simulink model "ROPOD_4Wheel_Tdistkinb_cntr_Code_GEN"  (R2017b)
settings: Solver=VariableStepAuto  StartTime=0.0  StopTime=10.0  RelTol=1e-3
values from neighbouring files (symbols this model uses):
  FFtheta_intia = 0    [init_model.m]
  FFxy_mass = 0*80    (= 0)    [init_model.m]
  I_fhz_dtheta_cntr = 0.3    [init_model.m]
  I_fhz_dvarphi_cntr = 0    [init_model.m]
  I_fhz_dxdy_cntr = 0.25    [init_model.m]
  K_gain_dtheta_cntr = 100    [init_model.m]
  K_gain_dvarphi_cntr = 0.03    [init_model.m]
  K_gain_dxdy_cntr = 150    [init_model.m]
  LL_wp_fhz_dtheta_cntr = 20    [init_model.m]
  LL_wp_fhz_dvarphi_cntr = 10    [init_model.m]
  LL_wp_fhz_dxdy_cntr = 20    [init_model.m]
  LL_wz_fhz_dtheta_cntr = 20    [init_model.m]
  LL_wz_fhz_dvarphi_cntr = 5    [init_model.m]
  LL_wz_fhz_dxdy_cntr = 20    [init_model.m]
  LPF_fhz_ddelta_meas = 50    [init_model.m]
  LPF_fhz_dtheta_cntr = 100    [init_model.m]
  LPF_fhz_dvarphi_cntr = 40    [init_model.m]
  LPF_fhz_dvarphi_meas = 50    [init_model.m]
  LPF_fhz_dxdy_cntr = 100    [init_model.m]
  max_hw_tau = 7.0    (= 7)    [init_model.m]
  max_ropod_acc_theta = 2.0    (= 2)    [init_model.m]
  max_ropod_acc_xy = 10.5    [init_model.m]
  max_ropod_vel_theta = 1.6    [init_model.m]
  max_ropod_vel_xy = 5.0    (= 5)    [init_model.m]
  max_sw_current = 15    [init_model.m]
  Nwheels = 4    [Jqwl_numeric_function.m]    (also in S_matrix.m; extract_kinmodel_parameters.m; init_model.m; tau_optimal_dist_vec_fun.m)
  pivot_offs_sws = 0*[3.835 3.465 2.059 0.357]    [init_model.m]
  ropod_kinmodel_pv = struct2array(ropod_kinmodel_param)    [set_ropod_KinModparams.m]
  SW_COM1_ENABLE1 = hex2dec('0001')    [init_model.m]
  SW_COM1_ENABLE2 = hex2dec('0002')    [init_model.m]
  SW_COM1_MODE_TORQUE = bitshift(hex2dec('0000'),2)    [init_model.m]
  SW_COM1_MODE_VELOCITY = bitshift(hex2dec('0002'),2)    [init_model.m]
  SW_COM1_USE_TS = hex2dec('8000')    [init_model.m]
  sw_tau_2_curr = 1/motor_physical_parameters.torqueconstant.value    [init_model.m]
  Tinit = 1*Tslot    [init_model.m]
  Ts = 0.001    [init_model.m]
undefined symbols (not defined in the file or in its folder): DiscIntNeverNeededParam
libraries: simulink x50, cstblocks x23, dspsigops x12, SOEM_EtherCAT_Lib x5
(part 1 of 4)
settings Model: Creator=cesar  LastModifiedBy=cesar
settings OptimizationCC: DefaultParameterBehavior=Inlined  UseFloatMulNetSlope=on  InlineInvariantSignals=on  EfficientFloat2IntCast=on
settings DebuggingCC: UnderSpecifiedDataTypeMsg=warning
settings HardwareCC: ProdBitPerLong=64  ProdHWDeviceType=Intel->x86-64 (Linux 64)
settings RTWCC: GenCodeOnly=on  BuildConfiguration=Faster Runs
settings GRTTargetCC: MatFileLogging=off  SupportNonFinite=off

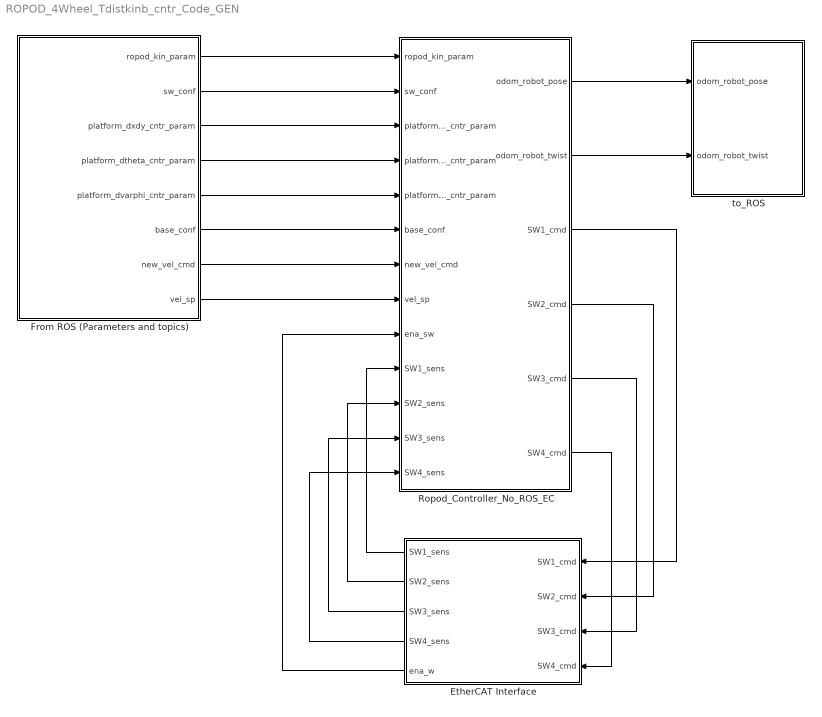
== system ROPOD_4Wheel_Tdistkinb_cntr_Code_GEN ==
  EtherCAT Interface : Subsystem
  From ROS (Parameters and topics) : Subsystem
  Ropod_Controller_No_ROS_EC : Subsystem
  to_ROS : Subsystem
  wires:
  From ROS (Parameters and topics)/1(ropod_kin_param) -> Ropod_Controller_No_ROS_EC/1(ropod_kin_param)
  Ropod_Controller_No_ROS_EC/6(SW4_cmd) -> EtherCAT Interface/4(SW4_cmd)
  From ROS (Parameters and topics)/4(platform_dtheta_cntr_param) -> Ropod_Controller_No_ROS_EC/4(platform_dtheta_cntr_param)
  Ropod_Controller_No_ROS_EC/3(SW1_cmd) -> EtherCAT Interface/1(SW1_cmd)
  From ROS (Parameters and topics)/3(platform_dxdy_cntr_param) -> Ropod_Controller_No_ROS_EC/3(platform_dxdy_cntr_param)
  Ropod_Controller_No_ROS_EC/4(SW2_cmd) -> EtherCAT Interface/2(SW2_cmd)
  EtherCAT Interface/4(SW4_sens) -> Ropod_Controller_No_ROS_EC/13(SW4_sens)
  Ropod_Controller_No_ROS_EC/2(odom_robot_twist) -> to_ROS/2(odom_robot_twist)
  Ropod_Controller_No_ROS_EC/5(SW3_cmd) -> EtherCAT Interface/3(SW3_cmd)
  From ROS (Parameters and topics)/8(vel_sp) -> Ropod_Controller_No_ROS_EC/8(vel_sp)
  From ROS (Parameters and topics)/6(base_conf) -> Ropod_Controller_No_ROS_EC/6(base_conf)
  EtherCAT Interface/1(SW1_sens) -> Ropod_Controller_No_ROS_EC/10(SW1_sens)
  From ROS (Parameters and topics)/2(sw_conf) -> Ropod_Controller_No_ROS_EC/2(sw_conf)
  From ROS (Parameters and topics)/5(platform_dvarphi_cntr_param) -> Ropod_Controller_No_ROS_EC/5(platform_dvarphi_cntr_param)
  EtherCAT Interface/2(SW2_sens) -> Ropod_Controller_No_ROS_EC/11(SW2_sens)
  EtherCAT Interface/5(ena_w) -> Ropod_Controller_No_ROS_EC/9(ena_sw)
  EtherCAT Interface/3(SW3_sens) -> Ropod_Controller_No_ROS_EC/12(SW3_sens)
  Ropod_Controller_No_ROS_EC/1(odom_robot_pose) -> to_ROS/1(odom_robot_pose)
  From ROS (Parameters and topics)/7(new_vel_cmd) -> Ropod_Controller_No_ROS_EC/7(new_vel_cmd)

== system ROPOD_4Wheel_Tdistkinb_cntr_Code_GEN/EtherCAT Interface ==
  SW1_cmd : Inport
  SW2_cmd : Inport  Port=2
  SW3_cmd : Inport  Port=3
  SW4_cmd : Inport  Port=4
  Constant : Constant  Value=[1 1 1 1]
  Display1 : Display  Commented=on
  ECAT_Interface : SOEM_EtherCAT_Lib/ECAT_Interface  Priority=0  Commented=on  IFINTERFACE=eth0  TS=Ts
      settings: SourceProductName=SOEM_EtherCAT_Lib
  Gain1 : Gain  Commented=on  OutDataTypeStr=double
  Smart_Wheel_1 : Subsystem
  Smart_Wheel_2 : Subsystem
  Smart_Wheel_3 : Subsystem
  Smart_Wheel_4 : Subsystem
  SW1_sens : Outport
  SW2_sens : Outport  Port=2
  SW3_sens : Outport  Port=3
  SW4_sens : Outport  Port=4
  ena_w : Outport  Port=5
  wires:
  Smart_Wheel_2/1(SW2_sens) -> SW2_sens/1  "SW2_sens"
  Smart_Wheel_3/1(SW3_sens) -> SW3_sens/1  "SW3_sens"
  SW4_cmd/1 -> Smart_Wheel_4/1(SW4_cmd)
  SW2_cmd/1 -> Smart_Wheel_2/1(SW2_cmd)
  SW3_cmd/1 -> Smart_Wheel_3/1(SW3_cmd)
  SW1_cmd/1 -> Smart_Wheel_1/1(SW1_cmd)
  Smart_Wheel_1/1(SW1_sens) -> SW1_sens/1  "SW1_sens"
  Smart_Wheel_4/1(SW4_sens) -> SW4_sens/1  "SW4_sens"
  ECAT_Interface/1 -> Gain1/1
  Gain1/1 -> Display1/1
  Constant/1 -> ena_w/1

== system ROPOD_4Wheel_Tdistkinb_cntr_Code_GEN/From ROS (Parameters and topics) ==
  note: doing the transformation with the angle from odometry data helps
      | to keep the robot better align during the Identification, especially because
      | we do not have any absolute reference
  Constant1 : Constant
  Controllers conf : Subsystem
  From Workspace1 : FromWorkspace  VariableName=qrefdot  SampleTime=0
  Gain1 : Gain
  ROS base conf : Subsystem
  Ropod kinematic parameters : Subsystem
  Selector1 : Selector  InputPortWidth=3  IndexOptions=Index vector (dialog)  Indices=3  OutputSizes=1
  Smart wheels conf1 : Subsystem
  rot_matrix2 : MATLAB Function  TreatAsAtomicUnit=on
  ropod_kin_param : Outport
  sw_conf : Outport  Port=2
  platform_dxdy_cntr_param : Outport  Port=3
  platform_dtheta_cntr_param : Outport  Port=4
  platform_dvarphi_cntr_param : Outport  Port=5
  base_conf : Outport  Port=6
  new_vel_cmd : Outport  Port=7
  vel_sp : Outport  Port=8
  wires:
  Controllers conf/1(platform_dxdy_cntr_param) -> platform_dxdy_cntr_param/1
  Constant1/1 -> new_vel_cmd/1
  Ropod kinematic parameters/1(ropod_kin_param) -> ropod_kin_param/1
  Gain1/1 -> vel_sp/1
  ROS base conf/1(base_conf) -> base_conf/1
  From Workspace1/1 -> Selector1/1, rot_matrix2/1(dqr_glb)
  Controllers conf/3(platform_dvarphi_cntr_param) -> platform_dvarphi_cntr_param/1
  Smart wheels conf1/1(sw_conf) -> sw_conf/1
  Controllers conf/2(platform_dtheta_cntr_param) -> platform_dtheta_cntr_param/1
  Selector1/1 -> rot_matrix2/2(theta)
  rot_matrix2/1(dqr_loc) -> Gain1/1

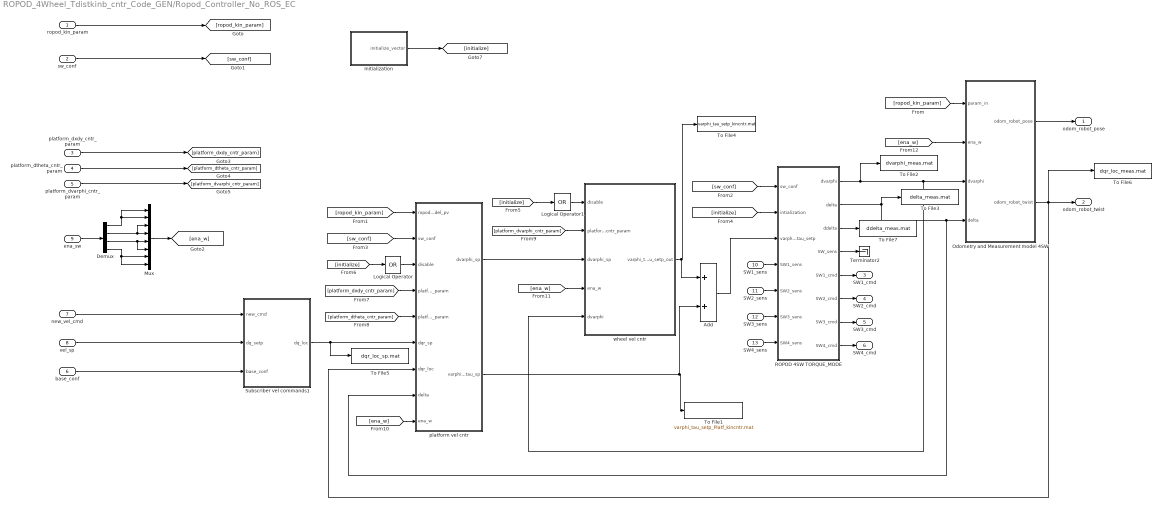
== system ROPOD_4Wheel_Tdistkinb_cntr_Code_GEN/Ropod_Controller_No_ROS_EC ==
  ropod_kin_param : Inport
  sw_conf : Inport  Port=2
  platform_dxdy_cntr_param : Inport  Port=3
  platform_dtheta_cntr_param : Inport  Port=4
  platform_dvarphi_cntr_param : Inport  Port=5
  base_conf : Inport  Port=6
  new_vel_cmd : Inport  Port=7
  vel_sp : Inport  Port=8
  ena_sw : Inport  Port=9
  SW1_sens : Inport  Port=10
  SW2_sens : Inport  Port=11
  SW3_sens : Inport  Port=12
  SW4_sens : Inport  Port=13
  Add : Sum
  Demux : Demux
  Initialization : Subsystem
  Logical Operator : Logic  Operator=OR  Inputs=1  AllPortsSameDT=off  OutDataTypeStr=boolean
  Logical Operator1 : Logic  Operator=OR  Inputs=1  AllPortsSameDT=off  OutDataTypeStr=boolean
  Mux : Mux  Inputs=8
  Odometry and Measurement model 4SW : Subsystem
  ROPOD 4SW TORQUE_MODE : Subsystem
  Subscriber vel commands1 : Subsystem
  Terminator2 : Terminator
  To File1 : ToFile  Filename=varphi_tau_setp_Platf_kincntr.mat  MatrixName=varphi_tau_setp_Platf_kincntr
  To File2 : ToFile  Filename=dvarphi_meas.mat  MatrixName=dvarphi_meas
  To File3 : ToFile  Filename=delta_meas.mat  MatrixName=delta_meas
  To File4 : ToFile  Filename=varphi_tau_setp_kincntr.mat  MatrixName=varphi_tau_setp_kincntr
  To File5 : ToFile  Filename=dqr_loc_sp.mat  MatrixName=dqr_loc_sp
  To File6 : ToFile  Filename=dqr_loc_meas.mat  MatrixName=dqr_loc_meas
  To File7 : ToFile  Filename=ddelta_meas.mat  MatrixName=ddelta_meas
  platform vel cntr : Subsystem
  wheel vel cntr : Subsystem
  odom_robot_pose : Outport
  odom_robot_twist : Outport  Port=2
  SW1_cmd : Outport  Port=3
  SW2_cmd : Outport  Port=4
  SW3_cmd : Outport  Port=5
  SW4_cmd : Outport  Port=6
  wires:
  sw_conf/1 -> [sw_conf]
  platform_dvarphi_cntr_param/1 -> [platform_dvarphi_cntr_param]
  platform_dxdy_cntr_param/1 -> [platform_dxdy_cntr_param]
  ropod_kin_param/1 -> [ropod_kin_param]
  platform_dtheta_cntr_param/1 -> [platform_dtheta_cntr_param]
  [ropod_kin_param] -> platform vel cntr/1(ropod_kinmodel_pv)
  ROPOD 4SW TORQUE_MODE/2(delta) -> To File3/1, platform vel cntr/8(delta), Odometry and Measurement model 4SW/4(delta)
  vel_sp/1 -> Subscriber vel commands1/2(dq_setp)
  ROPOD 4SW TORQUE_MODE/3(ddelta) -> To File7/1
  [initialize] -> Logical Operator/1
  wheel vel cntr/1(varphi_tau_setp_out) -> Add/1, To File4/1
  Odometry and Measurement model 4SW/2(odom_robot_twist) -> To File6/1, platform vel cntr/7(dqr_loc), odom_robot_twist/1
  [sw_conf] -> ROPOD 4SW TORQUE_MODE/1(sw_conf)
  platform vel cntr/1(dvarphi_sp) -> wheel vel cntr/3(dvarphi_sp)
  Subscriber vel commands1/1(dq_loc) -> To File5/1, platform vel cntr/6(dqr_sp)
  [platform_dvarphi_cntr_param] -> wheel vel cntr/2(platform_dxdy_cntr_param)
  base_conf/1 -> Subscriber vel commands1/3(base_conf)
  ROPOD 4SW TORQUE_MODE/1(dvarphi) -> To File2/1, wheel vel cntr/5(dvarphi), Odometry and Measurement model 4SW/3(dvarphi)
  [ropod_kin_param] -> Odometry and Measurement model 4SW/1(param_in)
  [ena_w] -> platform vel cntr/9(ena_w)
  Odometry and Measurement model 4SW/1(odom_robot_pose) -> odom_robot_pose/1
  new_vel_cmd/1 -> Subscriber vel commands1/1(new_cmd)
  [platform_dtheta_cntr_param] -> platform vel cntr/5(platform_dtheta_cntr_param)
  [initialize] -> Logical Operator1/1
  [platform_dxdy_cntr_param] -> platform vel cntr/4(platform_dxdy_cntr_param)
  [sw_conf] -> platform vel cntr/2(sw_conf)
  [initialize] -> ROPOD 4SW TORQUE_MODE/2(intialization)
  platform vel cntr/2(varphi_tau_sp) -> Add/2, To File1/1
  Initialization/1(initialize_vector) -> [initialize]
  Logical Operator/1 -> platform vel cntr/3(disable)
  Logical Operator1/1 -> wheel vel cntr/1(disable)
  [ena_w] -> wheel vel cntr/4(ena_w)
  [ena_w] -> Odometry and Measurement model 4SW/2(ena_w)
  ROPOD 4SW TORQUE_MODE/4(SW_sens) -> Terminator2/1
  ROPOD 4SW TORQUE_MODE/5(SW1_cmd) -> SW1_cmd/1
  ROPOD 4SW TORQUE_MODE/6(SW2_cmd) -> SW2_cmd/1
  ROPOD 4SW TORQUE_MODE/7(SW3_cmd) -> SW3_cmd/1
  ROPOD 4SW TORQUE_MODE/8(SW4_cmd) -> SW4_cmd/1
  SW1_sens/1 -> ROPOD 4SW TORQUE_MODE/4(SW1_sens)
  SW2_sens/1 -> ROPOD 4SW TORQUE_MODE/5(SW2_sens)
  SW3_sens/1 -> ROPOD 4SW TORQUE_MODE/6(SW3_sens)
  SW4_sens/1 -> ROPOD 4SW TORQUE_MODE/7(SW4_sens)
  ena_sw/1 -> Demux/1
  Demux/1 -> Mux/2, Mux/1
  Demux/2 -> Mux/3, Mux/4
  Demux/3 -> Mux/6, Mux/5
  Demux/4 -> Mux/7, Mux/8
  Mux/1 -> [ena_w]
  Add/1 -> ROPOD 4SW TORQUE_MODE/3(varphi_tau_setp)

== system ROPOD_4Wheel_Tdistkinb_cntr_Code_GEN/to_ROS ==
  odom_robot_pose : Inport
  odom_robot_twist : Inport  Port=2
  Terminator1 : Terminator
  Terminator2 : Terminator
  wires:
  odom_robot_pose/1 -> Terminator2/1
  odom_robot_twist/1 -> Terminator1/1

== system ROPOD_4Wheel_Tdistkinb_cntr_Code_GEN/EtherCAT Interface/Smart_Wheel_1 ==
  SW1_cmd : Inport
  Bus Creator1 : BusCreator  Inputs=40
  Bus Selector : BusSelector  OutputSignals=command1,command2,setpoint1,setpoint2,limit1_p,limit1_n,limit2_p,limit2_n,timestamp
  ec_ROPOD_SmartWheel : SOEM_EtherCAT_Lib/ec_ROPOD_SmartWheel  link_id=1
      settings: SourceProductName=SOEM_EtherCAT_Lib
  SW1_sens : Outport
  wires:
  Bus Creator1/1 -> SW1_sens/1
  ec_ROPOD_SmartWheel/21 -> Bus Creator1/21  "current_2_u"
  ec_ROPOD_SmartWheel/3 -> Bus Creator1/3  "sensor_ts"
  ec_ROPOD_SmartWheel/34 -> Bus Creator1/34  "accel_y"
  ec_ROPOD_SmartWheel/29 -> Bus Creator1/29  "encoder_pivot"
  ec_ROPOD_SmartWheel/18 -> Bus Creator1/18  "velocity_2"
  ec_ROPOD_SmartWheel/19 -> Bus Creator1/19  "current_2_d"
  ec_ROPOD_SmartWheel/14 -> Bus Creator1/14  "voltage_1_v"
  ec_ROPOD_SmartWheel/6 -> Bus Creator1/6  "velocity_1"
  ec_ROPOD_SmartWheel/12 -> Bus Creator1/12  "voltage_1"
  ec_ROPOD_SmartWheel/35 -> Bus Creator1/35  "accel_z"
  ec_ROPOD_SmartWheel/2 -> Bus Creator1/2  "status2"
  ec_ROPOD_SmartWheel/1 -> Bus Creator1/1  "status1"
  ec_ROPOD_SmartWheel/22 -> Bus Creator1/22  "current_2_v"
  ec_ROPOD_SmartWheel/25 -> Bus Creator1/25  "voltage_2_u"
  ec_ROPOD_SmartWheel/24 -> Bus Creator1/24  "voltage_2"
  ec_ROPOD_SmartWheel/15 -> Bus Creator1/15  "voltage_1_w"
  ec_ROPOD_SmartWheel/9 -> Bus Creator1/9  "current_1_u"
  ec_ROPOD_SmartWheel/28 -> Bus Creator1/28  "temperature_2"
  ec_ROPOD_SmartWheel/37 -> Bus Creator1/37  "gyro_y"
  ec_ROPOD_SmartWheel/20 -> Bus Creator1/20  "current_2_q"
  ec_ROPOD_SmartWheel/38 -> Bus Creator1/38  "gyro_z"
  ec_ROPOD_SmartWheel/13 -> Bus Creator1/13  "voltage_1_u"
  ec_ROPOD_SmartWheel/27 -> Bus Creator1/27  "voltage_2_w"
  ec_ROPOD_SmartWheel/7 -> Bus Creator1/7  "current_1_d"
  ec_ROPOD_SmartWheel/5 -> Bus Creator1/5  "encoder_1"
  ec_ROPOD_SmartWheel/36 -> Bus Creator1/36  "gyro_x"
  ec_ROPOD_SmartWheel/23 -> Bus Creator1/23  "current_2_w"
  ec_ROPOD_SmartWheel/4 -> Bus Creator1/4  "setpoint_ts"
  ec_ROPOD_SmartWheel/17 -> Bus Creator1/17  "encoder_2"
  ec_ROPOD_SmartWheel/11 -> Bus Creator1/11  "current_1_w"
  ec_ROPOD_SmartWheel/40 -> Bus Creator1/40  "pressure"
  ec_ROPOD_SmartWheel/30 -> Bus Creator1/30  "velocity_pivot"
  ec_ROPOD_SmartWheel/10 -> Bus Creator1/10  "current_1_v"
  ec_ROPOD_SmartWheel/39 -> Bus Creator1/39  "temperature_imu"
  ec_ROPOD_SmartWheel/16 -> Bus Creator1/16  "temperature_1"
  ec_ROPOD_SmartWheel/33 -> Bus Creator1/33  "accel_x"
  ec_ROPOD_SmartWheel/26 -> Bus Creator1/26  "voltage_2_v"
  ec_ROPOD_SmartWheel/8 -> Bus Creator1/8  "current_1_q"
  ec_ROPOD_SmartWheel/31 -> Bus Creator1/31  "voltage_bus"
  ec_ROPOD_SmartWheel/32 -> Bus Creator1/32  "imu_ts"
  SW1_cmd/1 -> Bus Selector/1
  Bus Selector/1 -> ec_ROPOD_SmartWheel/1  "<command1>"
  Bus Selector/2 -> ec_ROPOD_SmartWheel/2  "<command2>"
  Bus Selector/3 -> ec_ROPOD_SmartWheel/3  "<setpoint1>"
  Bus Selector/4 -> ec_ROPOD_SmartWheel/4  "<setpoint2>"
  Bus Selector/5 -> ec_ROPOD_SmartWheel/5  "<limit1_p>"
  Bus Selector/6 -> ec_ROPOD_SmartWheel/6  "<limit1_n>"
  Bus Selector/7 -> ec_ROPOD_SmartWheel/7  "<limit2_p>"
  Bus Selector/8 -> ec_ROPOD_SmartWheel/8  "<limit2_n>"
  Bus Selector/9 -> ec_ROPOD_SmartWheel/9  "<timestamp>"

== system ROPOD_4Wheel_Tdistkinb_cntr_Code_GEN/EtherCAT Interface/Smart_Wheel_2 ==
  SW2_cmd : Inport
  Bus Creator1 : BusCreator  Inputs=40
  Bus Selector : BusSelector  OutputSignals=command1,command2,setpoint1,setpoint2,limit1_p,limit1_n,limit2_p,limit2_n,timestamp
  ec_ROPOD_SmartWheel : SOEM_EtherCAT_Lib/ec_ROPOD_SmartWheel  link_id=2
      settings: SourceProductName=SOEM_EtherCAT_Lib
  SW2_sens : Outport
  wires:
  Bus Selector/9 -> ec_ROPOD_SmartWheel/9  "<timestamp>"
  Bus Selector/8 -> ec_ROPOD_SmartWheel/8  "<limit2_n>"
  Bus Selector/7 -> ec_ROPOD_SmartWheel/7  "<limit2_p>"
  Bus Selector/6 -> ec_ROPOD_SmartWheel/6  "<limit1_n>"
  Bus Selector/5 -> ec_ROPOD_SmartWheel/5  "<limit1_p>"
  Bus Selector/4 -> ec_ROPOD_SmartWheel/4  "<setpoint2>"
  Bus Selector/3 -> ec_ROPOD_SmartWheel/3  "<setpoint1>"
  Bus Selector/2 -> ec_ROPOD_SmartWheel/2  "<command2>"
  Bus Selector/1 -> ec_ROPOD_SmartWheel/1  "<command1>"
  SW2_cmd/1 -> Bus Selector/1
  ec_ROPOD_SmartWheel/32 -> Bus Creator1/32  "imu_ts"
  ec_ROPOD_SmartWheel/31 -> Bus Creator1/31  "voltage_bus"
  ec_ROPOD_SmartWheel/8 -> Bus Creator1/8  "current_1_q"
  ec_ROPOD_SmartWheel/26 -> Bus Creator1/26  "voltage_2_v"
  ec_ROPOD_SmartWheel/33 -> Bus Creator1/33  "accel_x"
  ec_ROPOD_SmartWheel/16 -> Bus Creator1/16  "temperature_1"
  ec_ROPOD_SmartWheel/39 -> Bus Creator1/39  "temperature_imu"
  ec_ROPOD_SmartWheel/10 -> Bus Creator1/10  "current_1_v"
  ec_ROPOD_SmartWheel/30 -> Bus Creator1/30  "velocity_pivot"
  ec_ROPOD_SmartWheel/40 -> Bus Creator1/40  "pressure"
  ec_ROPOD_SmartWheel/11 -> Bus Creator1/11  "current_1_w"
  ec_ROPOD_SmartWheel/17 -> Bus Creator1/17  "encoder_2"
  ec_ROPOD_SmartWheel/4 -> Bus Creator1/4  "setpoint_ts"
  ec_ROPOD_SmartWheel/23 -> Bus Creator1/23  "current_2_w"
  ec_ROPOD_SmartWheel/36 -> Bus Creator1/36  "gyro_x"
  ec_ROPOD_SmartWheel/5 -> Bus Creator1/5  "encoder_1"
  ec_ROPOD_SmartWheel/7 -> Bus Creator1/7  "current_1_d"
  ec_ROPOD_SmartWheel/27 -> Bus Creator1/27  "voltage_2_w"
  ec_ROPOD_SmartWheel/13 -> Bus Creator1/13  "voltage_1_u"
  ec_ROPOD_SmartWheel/38 -> Bus Creator1/38  "gyro_z"
  ec_ROPOD_SmartWheel/20 -> Bus Creator1/20  "current_2_q"
  ec_ROPOD_SmartWheel/37 -> Bus Creator1/37  "gyro_y"
  ec_ROPOD_SmartWheel/28 -> Bus Creator1/28  "temperature_2"
  ec_ROPOD_SmartWheel/9 -> Bus Creator1/9  "current_1_u"
  ec_ROPOD_SmartWheel/15 -> Bus Creator1/15  "voltage_1_w"
  ec_ROPOD_SmartWheel/24 -> Bus Creator1/24  "voltage_2"
  ec_ROPOD_SmartWheel/25 -> Bus Creator1/25  "voltage_2_u"
  ec_ROPOD_SmartWheel/22 -> Bus Creator1/22  "current_2_v"
  ec_ROPOD_SmartWheel/1 -> Bus Creator1/1  "status1"
  ec_ROPOD_SmartWheel/2 -> Bus Creator1/2  "status2"
  ec_ROPOD_SmartWheel/35 -> Bus Creator1/35  "accel_z"
  ec_ROPOD_SmartWheel/12 -> Bus Creator1/12  "voltage_1"
  ec_ROPOD_SmartWheel/6 -> Bus Creator1/6  "velocity_1"
  ec_ROPOD_SmartWheel/14 -> Bus Creator1/14  "voltage_1_v"
  ec_ROPOD_SmartWheel/19 -> Bus Creator1/19  "current_2_d"
  ec_ROPOD_SmartWheel/18 -> Bus Creator1/18  "velocity_2"
  ec_ROPOD_SmartWheel/29 -> Bus Creator1/29  "encoder_pivot"
  ec_ROPOD_SmartWheel/34 -> Bus Creator1/34  "accel_y"
  ec_ROPOD_SmartWheel/3 -> Bus Creator1/3  "sensor_ts"
  ec_ROPOD_SmartWheel/21 -> Bus Creator1/21  "current_2_u"
  Bus Creator1/1 -> SW2_sens/1

== system ROPOD_4Wheel_Tdistkinb_cntr_Code_GEN/EtherCAT Interface/Smart_Wheel_3 ==
  SW3_cmd : Inport
  Bus Creator1 : BusCreator  Inputs=40
  Bus Selector : BusSelector  OutputSignals=command1,command2,setpoint1,setpoint2,limit1_p,limit1_n,limit2_p,limit2_n,timestamp
  ec_ROPOD_SmartWheel : SOEM_EtherCAT_Lib/ec_ROPOD_SmartWheel  link_id=3
      settings: SourceProductName=SOEM_EtherCAT_Lib
  SW3_sens : Outport
  wires:
  Bus Creator1/1 -> SW3_sens/1
  ec_ROPOD_SmartWheel/21 -> Bus Creator1/21  "current_2_u"
  ec_ROPOD_SmartWheel/3 -> Bus Creator1/3  "sensor_ts"
  ec_ROPOD_SmartWheel/34 -> Bus Creator1/34  "accel_y"
  ec_ROPOD_SmartWheel/29 -> Bus Creator1/29  "encoder_pivot"
  ec_ROPOD_SmartWheel/18 -> Bus Creator1/18  "velocity_2"
  ec_ROPOD_SmartWheel/19 -> Bus Creator1/19  "current_2_d"
  ec_ROPOD_SmartWheel/14 -> Bus Creator1/14  "voltage_1_v"
  ec_ROPOD_SmartWheel/6 -> Bus Creator1/6  "velocity_1"
  ec_ROPOD_SmartWheel/12 -> Bus Creator1/12  "voltage_1"
  ec_ROPOD_SmartWheel/35 -> Bus Creator1/35  "accel_z"
  ec_ROPOD_SmartWheel/2 -> Bus Creator1/2  "status2"
  ec_ROPOD_SmartWheel/1 -> Bus Creator1/1  "status1"
  ec_ROPOD_SmartWheel/22 -> Bus Creator1/22  "current_2_v"
  ec_ROPOD_SmartWheel/25 -> Bus Creator1/25  "voltage_2_u"
  ec_ROPOD_SmartWheel/24 -> Bus Creator1/24  "voltage_2"
  ec_ROPOD_SmartWheel/15 -> Bus Creator1/15  "voltage_1_w"
  ec_ROPOD_SmartWheel/9 -> Bus Creator1/9  "current_1_u"
  ec_ROPOD_SmartWheel/28 -> Bus Creator1/28  "temperature_2"
  ec_ROPOD_SmartWheel/37 -> Bus Creator1/37  "gyro_y"
  ec_ROPOD_SmartWheel/20 -> Bus Creator1/20  "current_2_q"
  ec_ROPOD_SmartWheel/38 -> Bus Creator1/38  "gyro_z"
  ec_ROPOD_SmartWheel/13 -> Bus Creator1/13  "voltage_1_u"
  ec_ROPOD_SmartWheel/27 -> Bus Creator1/27  "voltage_2_w"
  ec_ROPOD_SmartWheel/7 -> Bus Creator1/7  "current_1_d"
  ec_ROPOD_SmartWheel/5 -> Bus Creator1/5  "encoder_1"
  ec_ROPOD_SmartWheel/36 -> Bus Creator1/36  "gyro_x"
  ec_ROPOD_SmartWheel/23 -> Bus Creator1/23  "current_2_w"
  ec_ROPOD_SmartWheel/4 -> Bus Creator1/4  "setpoint_ts"
  ec_ROPOD_SmartWheel/17 -> Bus Creator1/17  "encoder_2"
  ec_ROPOD_SmartWheel/11 -> Bus Creator1/11  "current_1_w"
  ec_ROPOD_SmartWheel/40 -> Bus Creator1/40  "pressure"
  ec_ROPOD_SmartWheel/30 -> Bus Creator1/30  "velocity_pivot"
  ec_ROPOD_SmartWheel/10 -> Bus Creator1/10  "current_1_v"
  ec_ROPOD_SmartWheel/39 -> Bus Creator1/39  "temperature_imu"
  ec_ROPOD_SmartWheel/16 -> Bus Creator1/16  "temperature_1"
  ec_ROPOD_SmartWheel/33 -> Bus Creator1/33  "accel_x"
  ec_ROPOD_SmartWheel/26 -> Bus Creator1/26  "voltage_2_v"
  ec_ROPOD_SmartWheel/8 -> Bus Creator1/8  "current_1_q"
  ec_ROPOD_SmartWheel/31 -> Bus Creator1/31  "voltage_bus"
  ec_ROPOD_SmartWheel/32 -> Bus Creator1/32  "imu_ts"
  SW3_cmd/1 -> Bus Selector/1
  Bus Selector/1 -> ec_ROPOD_SmartWheel/1  "<command1>"
  Bus Selector/2 -> ec_ROPOD_SmartWheel/2  "<command2>"
  Bus Selector/3 -> ec_ROPOD_SmartWheel/3  "<setpoint1>"
  Bus Selector/4 -> ec_ROPOD_SmartWheel/4  "<setpoint2>"
  Bus Selector/5 -> ec_ROPOD_SmartWheel/5  "<limit1_p>"
  Bus Selector/6 -> ec_ROPOD_SmartWheel/6  "<limit1_n>"
  Bus Selector/7 -> ec_ROPOD_SmartWheel/7  "<limit2_p>"
  Bus Selector/8 -> ec_ROPOD_SmartWheel/8  "<limit2_n>"
  Bus Selector/9 -> ec_ROPOD_SmartWheel/9  "<timestamp>"

== system ROPOD_4Wheel_Tdistkinb_cntr_Code_GEN/EtherCAT Interface/Smart_Wheel_4 ==
  SW4_cmd : Inport
  Bus Creator1 : BusCreator  Inputs=40
  Bus Selector : BusSelector  OutputSignals=command1,command2,setpoint1,setpoint2,limit1_p,limit1_n,limit2_p,limit2_n,timestamp
  ec_ROPOD_SmartWheel : SOEM_EtherCAT_Lib/ec_ROPOD_SmartWheel  link_id=4
      settings: SourceProductName=SOEM_EtherCAT_Lib
  SW4_sens : Outport
  wires:
  Bus Selector/9 -> ec_ROPOD_SmartWheel/9  "<timestamp>"
  Bus Selector/8 -> ec_ROPOD_SmartWheel/8  "<limit2_n>"
  Bus Selector/7 -> ec_ROPOD_SmartWheel/7  "<limit2_p>"
  Bus Selector/6 -> ec_ROPOD_SmartWheel/6  "<limit1_n>"
  Bus Selector/5 -> ec_ROPOD_SmartWheel/5  "<limit1_p>"
  Bus Selector/4 -> ec_ROPOD_SmartWheel/4  "<setpoint2>"
  Bus Selector/3 -> ec_ROPOD_SmartWheel/3  "<setpoint1>"
  Bus Selector/2 -> ec_ROPOD_SmartWheel/2  "<command2>"
  Bus Selector/1 -> ec_ROPOD_SmartWheel/1  "<command1>"
  SW4_cmd/1 -> Bus Selector/1
  ec_ROPOD_SmartWheel/32 -> Bus Creator1/32  "imu_ts"
  ec_ROPOD_SmartWheel/31 -> Bus Creator1/31  "voltage_bus"
  ec_ROPOD_SmartWheel/8 -> Bus Creator1/8  "current_1_q"
  ec_ROPOD_SmartWheel/26 -> Bus Creator1/26  "voltage_2_v"
  ec_ROPOD_SmartWheel/33 -> Bus Creator1/33  "accel_x"
  ec_ROPOD_SmartWheel/16 -> Bus Creator1/16  "temperature_1"
  ec_ROPOD_SmartWheel/39 -> Bus Creator1/39  "temperature_imu"
  ec_ROPOD_SmartWheel/10 -> Bus Creator1/10  "current_1_v"
  ec_ROPOD_SmartWheel/30 -> Bus Creator1/30  "velocity_pivot"
  ec_ROPOD_SmartWheel/40 -> Bus Creator1/40  "pressure"
  ec_ROPOD_SmartWheel/11 -> Bus Creator1/11  "current_1_w"
  ec_ROPOD_SmartWheel/17 -> Bus Creator1/17  "encoder_2"
  ec_ROPOD_SmartWheel/4 -> Bus Creator1/4  "setpoint_ts"
  ec_ROPOD_SmartWheel/23 -> Bus Creator1/23  "current_2_w"
  ec_ROPOD_SmartWheel/36 -> Bus Creator1/36  "gyro_x"
  ec_ROPOD_SmartWheel/5 -> Bus Creator1/5  "encoder_1"
  ec_ROPOD_SmartWheel/7 -> Bus Creator1/7  "current_1_d"
  ec_ROPOD_SmartWheel/27 -> Bus Creator1/27  "voltage_2_w"
  ec_ROPOD_SmartWheel/13 -> Bus Creator1/13  "voltage_1_u"
  ec_ROPOD_SmartWheel/38 -> Bus Creator1/38  "gyro_z"
  ec_ROPOD_SmartWheel/20 -> Bus Creator1/20  "current_2_q"
  ec_ROPOD_SmartWheel/37 -> Bus Creator1/37  "gyro_y"
  ec_ROPOD_SmartWheel/28 -> Bus Creator1/28  "temperature_2"
  ec_ROPOD_SmartWheel/9 -> Bus Creator1/9  "current_1_u"
  ec_ROPOD_SmartWheel/15 -> Bus Creator1/15  "voltage_1_w"
  ec_ROPOD_SmartWheel/24 -> Bus Creator1/24  "voltage_2"
  ec_ROPOD_SmartWheel/25 -> Bus Creator1/25  "voltage_2_u"
  ec_ROPOD_SmartWheel/22 -> Bus Creator1/22  "current_2_v"
  ec_ROPOD_SmartWheel/1 -> Bus Creator1/1  "status1"
  ec_ROPOD_SmartWheel/2 -> Bus Creator1/2  "status2"
  ec_ROPOD_SmartWheel/35 -> Bus Creator1/35  "accel_z"
  ec_ROPOD_SmartWheel/12 -> Bus Creator1/12  "voltage_1"
  ec_ROPOD_SmartWheel/6 -> Bus Creator1/6  "velocity_1"
  ec_ROPOD_SmartWheel/14 -> Bus Creator1/14  "voltage_1_v"
  ec_ROPOD_SmartWheel/19 -> Bus Creator1/19  "current_2_d"
  ec_ROPOD_SmartWheel/18 -> Bus Creator1/18  "velocity_2"
  ec_ROPOD_SmartWheel/29 -> Bus Creator1/29  "encoder_pivot"
  ec_ROPOD_SmartWheel/34 -> Bus Creator1/34  "accel_y"
  ec_ROPOD_SmartWheel/3 -> Bus Creator1/3  "sensor_ts"
  ec_ROPOD_SmartWheel/21 -> Bus Creator1/21  "current_2_u"
  Bus Creator1/1 -> SW4_sens/1

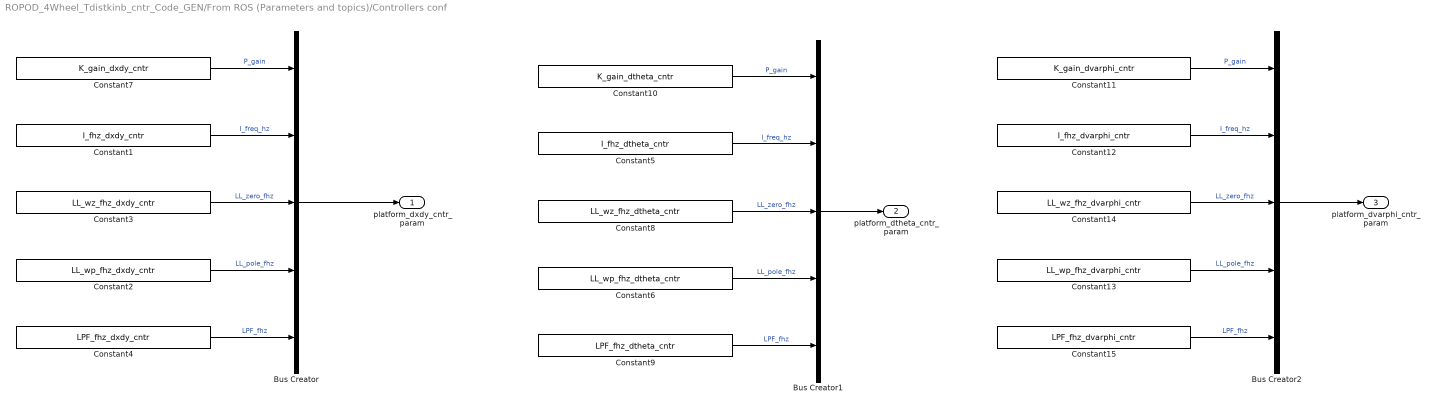
== system ROPOD_4Wheel_Tdistkinb_cntr_Code_GEN/From ROS (Parameters and topics)/Controllers conf ==
  Bus Creator : BusCreator  Inputs=5
  Bus Creator1 : BusCreator  Inputs=5
  Bus Creator2 : BusCreator  Inputs=5
  Constant1 : Constant  Value=I_fhz_dxdy_cntr
  Constant10 : Constant  Value=K_gain_dtheta_cntr
  Constant11 : Constant  Value=K_gain_dvarphi_cntr
  Constant12 : Constant  Value=I_fhz_dvarphi_cntr
  Constant13 : Constant  Value=LL_wp_fhz_dvarphi_cntr
  Constant14 : Constant  Value=LL_wz_fhz_dvarphi_cntr
  Constant15 : Constant  Value=LPF_fhz_dvarphi_cntr
  Constant2 : Constant  Value=LL_wp_fhz_dxdy_cntr
  Constant3 : Constant  Value=LL_wz_fhz_dxdy_cntr
  Constant4 : Constant  Value=LPF_fhz_dxdy_cntr
  Constant5 : Constant  Value=I_fhz_dtheta_cntr
  Constant6 : Constant  Value=LL_wp_fhz_dtheta_cntr
  Constant7 : Constant  Value=K_gain_dxdy_cntr
  Constant8 : Constant  Value=LL_wz_fhz_dtheta_cntr
  Constant9 : Constant  Value=LPF_fhz_dtheta_cntr
  platform_dxdy_cntr_param : Outport
  platform_dtheta_cntr_param : Outport  Port=2
  platform_dvarphi_cntr_param : Outport  Port=3
  wires:
  Constant2/1 -> Bus Creator/4  "LL_pole_fhz"
  Constant4/1 -> Bus Creator/5  "LPF_fhz"
  Bus Creator/1 -> platform_dxdy_cntr_param/1
  Constant1/1 -> Bus Creator/2  "I_freq_hz"
  Constant3/1 -> Bus Creator/3  "LL_zero_fhz"
  Constant7/1 -> Bus Creator/1  "P_gain"
  Bus Creator1/1 -> platform_dtheta_cntr_param/1
  Bus Creator2/1 -> platform_dvarphi_cntr_param/1
  Constant5/1 -> Bus Creator1/2  "I_freq_hz"
  Constant6/1 -> Bus Creator1/4  "LL_pole_fhz"
  Constant10/1 -> Bus Creator1/1  "P_gain"
  Constant8/1 -> Bus Creator1/3  "LL_zero_fhz"
  Constant9/1 -> Bus Creator1/5  "LPF_fhz"
  Constant15/1 -> Bus Creator2/5  "LPF_fhz"
  Constant12/1 -> Bus Creator2/2  "I_freq_hz"
  Constant14/1 -> Bus Creator2/3  "LL_zero_fhz"
  Constant11/1 -> Bus Creator2/1  "P_gain"
  Constant13/1 -> Bus Creator2/4  "LL_pole_fhz"

== system ROPOD_4Wheel_Tdistkinb_cntr_Code_GEN/From ROS (Parameters and topics)/ROS base conf ==
  Bus Creator : BusCreator  Inputs=4
  max_ropod_acc_theta : Constant  Value=max_ropod_acc_theta
  max_ropod_acc_xy : Constant  Value=max_ropod_acc_xy
  max_ropod_vel_theta : Constant  Value=max_ropod_vel_theta
  max_ropod_vel_xy : Constant  Value=max_ropod_vel_xy
  base_conf : Outport
  wires:
  max_ropod_acc_xy/1 -> Bus Creator/2  "max_acc_xy"
  max_ropod_vel_xy/1 -> Bus Creator/1  "max_vel_xy"
  Bus Creator/1 -> base_conf/1
  max_ropod_acc_theta/1 -> Bus Creator/4  "max_acc_theta"
  max_ropod_vel_theta/1 -> Bus Creator/3  "max_vel_theta"

== system ROPOD_4Wheel_Tdistkinb_cntr_Code_GEN/From ROS (Parameters and topics)/Ropod kinematic parameters ==
  ropod_kinmodel_pv : Constant  Value=ropod_kinmodel_pv
  ropod_kin_param : Outport
  wires:
  ropod_kinmodel_pv/1 -> ropod_kin_param/1

== system ROPOD_4Wheel_Tdistkinb_cntr_Code_GEN/From ROS (Parameters and topics)/Smart wheels conf1 ==
  Bus Creator : BusCreator  Inputs=8
  LPF_fhz_ddelta_meas : Constant  Value=LPF_fhz_ddelta_meas
  LPF_fhz_dvarphi_meas : Constant  Value=LPF_fhz_dvarphi_meas
  enable : Constant
  max_current : Constant  Value=max_sw_current
  pivot_offset_sw1 : Constant  Value=pivot_offs_sws(1)
  pivot_offset_sw2 : Constant  Value=pivot_offs_sws(2)
  pivot_offset_sw3 : Constant  Value=pivot_offs_sws(3)
  pivot_offset_sw4 : Constant  Value=pivot_offs_sws(4)
  sw_conf : Outport
  wires:
  enable/1 -> Bus Creator/1  "enable"
  Bus Creator/1 -> sw_conf/1
  max_current/1 -> Bus Creator/2  "max_current"
  pivot_offset_sw1/1 -> Bus Creator/3  "pivot_offs_sw1"
  pivot_offset_sw2/1 -> Bus Creator/4  "pivot_offs_sw2"
  pivot_offset_sw3/1 -> Bus Creator/5  "pivot_offs_sw3"
  pivot_offset_sw4/1 -> Bus Creator/6  "pivot_offs_sw4"
  LPF_fhz_dvarphi_meas/1 -> Bus Creator/7  "dvarphi_LPF_fhz"
  LPF_fhz_ddelta_meas/1 -> Bus Creator/8  "ddelta_LPF_fhz"

== system ROPOD_4Wheel_Tdistkinb_cntr_Code_GEN/Ropod_Controller_No_ROS_EC/Initialization ==
  note: Allow Tinit/Nwheels seconds for initialization per wheel
  Allow Tinit seconds for initialization : simulink/Logic and Bit Operations/Compare To Constant  relop=<  const=Tinit  OutDataTypeStr=boolean
  Digital Clock : DigitalClock  SampleTime=Ts
  Logical Operator : Logic  AllPortsSameDT=off  OutDataTypeStr=boolean
  Logical Operator1 : Logic  Operator=NOT  AllPortsSameDT=off  OutDataTypeStr=boolean
  Logical Operator2 : Logic  Operator=NOT  AllPortsSameDT=off  OutDataTypeStr=boolean
  Logical Operator3 : Logic  AllPortsSameDT=off  OutDataTypeStr=boolean
  Logical Operator4 : Logic  Operator=NOT  AllPortsSameDT=off  OutDataTypeStr=boolean
  Logical Operator5 : Logic  AllPortsSameDT=off  OutDataTypeStr=boolean
  Logical Operator{6..9} (4 alike) : Logic  Operator=OR  AllPortsSameDT=off  OutDataTypeStr=boolean
  Manual Switch : ManualSwitch  CurrentSetting=0
  Mux : Mux
  Mux1 : Mux
  comp : simulink/Logic and Bit Operations/Compare To Constant  relop=<  const=Tinit/Nwheels  OutDataTypeStr=boolean
  comp1 : simulink/Logic and Bit Operations/Compare To Constant  relop=<  const=2*Tinit/Nwheels  OutDataTypeStr=boolean
  comp2 : simulink/Logic and Bit Operations/Compare To Constant  relop=<  const=3*Tinit/Nwheels  OutDataTypeStr=boolean
  comp3 : simulink/Logic and Bit Operations/Compare To Constant  relop=<  const=4*Tinit/Nwheels  OutDataTypeStr=boolean
  initialize_vector : Outport
  wires:
  comp3/1 -> Logical Operator5/2
  Logical Operator2/1 -> Logical Operator3/1
  Logical Operator1/1 -> Logical Operator/1
  Logical Operator4/1 -> Logical Operator5/1
  comp/1 -> Logical Operator6/1, Mux/1, Logical Operator1/1
  comp1/1 -> Logical Operator2/1, Logical Operator/2
  comp2/1 -> Logical Operator4/1, Logical Operator3/2
  Digital Clock/1 -> Allow Tinit seconds for initialization/1, comp3/1, comp2/1, comp1/1, comp/1
  Logical Operator/1 -> Logical Operator7/1, Mux/2
  Logical Operator3/1 -> Logical Operator8/1, Mux/3
  Logical Operator5/1 -> Logical Operator9/1, Mux/4
  Logical Operator6/1 -> Mux1/1
  Logical Operator7/1 -> Mux1/2
  Logical Operator8/1 -> Mux1/3
  Logical Operator9/1 -> Mux1/4
  Allow Tinit seconds for initialization/1 -> Logical Operator6/2, Logical Operator7/2, Logical Operator8/2, Logical Operator9/2
  Manual Switch/1 -> initialize_vector/1
  Mux/1 -> Manual Switch/1
  Mux1/1 -> Manual Switch/2

== system ROPOD_4Wheel_Tdistkinb_cntr_Code_GEN/Ropod_Controller_No_ROS_EC/Odometry and Measurement model 4SW ==
  note: This output is only useful when using ros
      | This data is fed to /odom/pose
  note: This part is in global coordinates
  note: This part is in local coordinates
  param_in : Inport
  ena_w : Inport  Port=2
  dvarphi : Inport  Port=3
  delta : Inport  Port=4
  Discrete-Time Integrator : DiscreteIntegrator  InitialConditionSetting=State (most efficient)  SampleTime=Ts  ICPrevOutput=DiscIntNeverNeededParam  ICPrevScaledInput=DiscIntNeverNeededParam
  Jqwl_numeric : MATLAB Function  TreatAsAtomicUnit=on
  Selector3 : Selector  IndexMode=Zero-based  InputPortWidth=3  IndexOptions=Index vector (dialog)  Indices=2  OutputSizes=1
  Signal Specification : SignalSpecification  Dimensions=[3 1]
  pos_rot_matrix : MATLAB Function  TreatAsAtomicUnit=on
  odom_robot_pose : Outport
  odom_robot_twist : Outport  Port=2
  wires:
  Jqwl_numeric/1(v) -> Signal Specification/1
  param_in/1 -> Jqwl_numeric/1(ropod_kinmodel_param_vec)
  delta/1 -> Jqwl_numeric/2(delta)
  Signal Specification/1 -> pos_rot_matrix/1(dqr_loc), odom_robot_twist/1
  Selector3/1 -> pos_rot_matrix/2(theta_odom)
  pos_rot_matrix/1(dqr_glb) -> Discrete-Time Integrator/1
  Discrete-Time Integrator/1 -> odom_robot_pose/1, Selector3/1
  dvarphi/1 -> Jqwl_numeric/3(dvarphi)
  ena_w/1 -> Jqwl_numeric/4(ena_w)

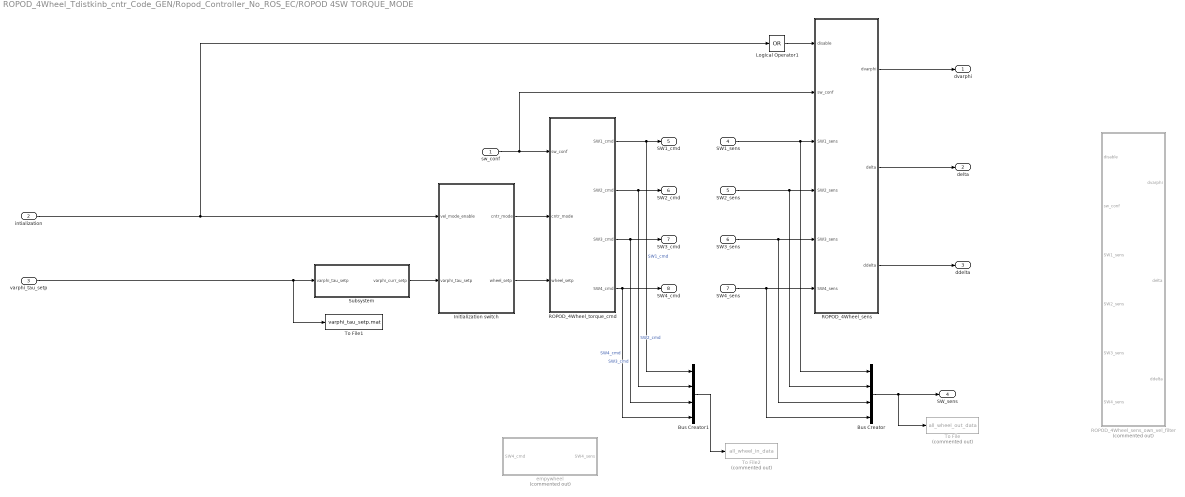
== system ROPOD_4Wheel_Tdistkinb_cntr_Code_GEN/Ropod_Controller_No_ROS_EC/ROPOD 4SW TORQUE_MODE ==
  sw_conf : Inport
  intialization : Inport  Port=2
  varphi_tau_setp : Inport  Port=3
  SW1_sens : Inport  Port=4
  SW2_sens : Inport  Port=5
  SW3_sens : Inport  Port=6
  SW4_sens : Inport  Port=7
  Bus Creator : BusCreator  Inputs=4
  Bus Creator1 : BusCreator  Inputs=4
  Initialization switch : Subsystem
  Logical Operator1 : Logic  Operator=OR  Inputs=1  AllPortsSameDT=off  OutDataTypeStr=boolean
  ROPOD_4Wheel_sens : Subsystem
  ROPOD_4Wheel_sens_own_vel_filter : Subsystem  Commented=on
  ROPOD_4Wheel_torque_cmd : Subsystem
  Subsystem : Subsystem
  To File : ToFile  Commented=on  Filename=all_wheel_out_data  MatrixName=all_wheel_out_data
  To File1 : ToFile  Filename=varphi_tau_setp.mat  MatrixName=varphi_tau_setp
  To File2 : ToFile  Commented=on  Filename=all_wheel_in_data  MatrixName=all_wheel_in_data
  empywheel : Subsystem  Commented=on
  dvarphi : Outport
  delta : Outport  Port=2
  ddelta : Outport  Port=3
  SW_sens : Outport  Port=4
  SW1_cmd : Outport  Port=5
  SW2_cmd : Outport  Port=6
  SW3_cmd : Outport  Port=7
  SW4_cmd : Outport  Port=8
  wires:
  ROPOD_4Wheel_sens/2(delta) -> delta/1
  ROPOD_4Wheel_sens/1(dvarphi) -> dvarphi/1
  ROPOD_4Wheel_sens/3(ddelta) -> ddelta/1
  ROPOD_4Wheel_torque_cmd/4(SW4_cmd) -> SW4_cmd/1, Bus Creator1/4  "SW4_cmd"
  ROPOD_4Wheel_torque_cmd/1(SW1_cmd) -> SW1_cmd/1, Bus Creator1/1  "SW1_cmd"
  ROPOD_4Wheel_torque_cmd/3(SW3_cmd) -> SW3_cmd/1, Bus Creator1/3  "SW3_cmd"
  sw_conf/1 -> ROPOD_4Wheel_sens/2(sw_conf), ROPOD_4Wheel_torque_cmd/1(sw_conf)
  ROPOD_4Wheel_torque_cmd/2(SW2_cmd) -> SW2_cmd/1, Bus Creator1/2  "SW2_cmd"
  Bus Creator/1 -> To File/1, SW_sens/1
  Initialization switch/1(cntr_mode) -> ROPOD_4Wheel_torque_cmd/2(cntr_mode)
  Initialization switch/2(wheel_setp) -> ROPOD_4Wheel_torque_cmd/3(wheel_setp)
  Subsystem/1(varphi_curr_setp) -> Initialization switch/2(varphi_tau_setp)
  varphi_tau_setp/1 -> To File1/1, Subsystem/1(varphi_tau_setp)
  intialization/1 -> Initialization switch/1(vel_mode_enable), Logical Operator1/1
  Bus Creator1/1 -> To File2/1
  SW3_sens/1 -> ROPOD_4Wheel_sens/5(SW3_sens), Bus Creator/3
  SW2_sens/1 -> ROPOD_4Wheel_sens/4(SW2_sens), Bus Creator/2
  SW4_sens/1 -> ROPOD_4Wheel_sens/6(SW4_sens), Bus Creator/4
  SW1_sens/1 -> ROPOD_4Wheel_sens/3(SW1_sens), Bus Creator/1
  Logical Operator1/1 -> ROPOD_4Wheel_sens/1(disable)

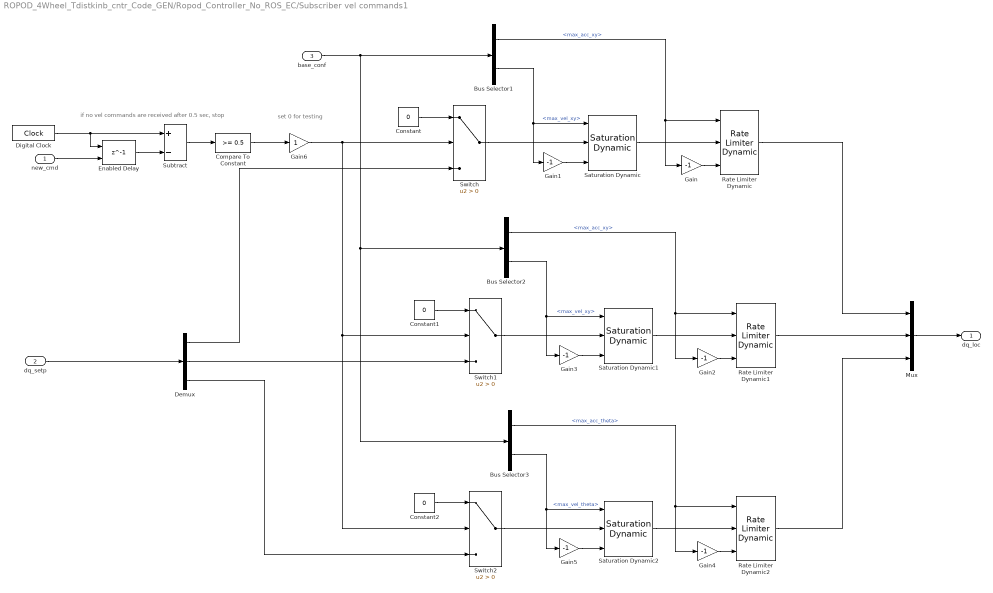
== system ROPOD_4Wheel_Tdistkinb_cntr_Code_GEN/Ropod_Controller_No_ROS_EC/Subscriber vel commands1 ==
  note: set 0 for testing
  note: if no vel commands are received after 0.5 sec, stop
  new_cmd : Inport
  dq_setp : Inport  Port=2
  base_conf : Inport  Port=3
  Bus Selector1 : BusSelector  OutputSignals=max_acc_xy,max_vel_xy
  Bus Selector2 : BusSelector  OutputSignals=max_acc_xy,max_vel_xy
  Bus Selector3 : BusSelector  OutputSignals=max_acc_theta,max_vel_theta
  Compare To Constant : simulink/Logic and Bit Operations/Compare To Constant  relop=>=  const=0.5  OutDataTypeStr=boolean
  Constant : Constant  Value=0  SampleTime=Ts
  Constant1 : Constant  Value=0
  Constant2 : Constant  Value=0
  Demux : Demux  Outputs=3
  Digital Clock : DigitalClock  SampleTime=Ts
  Enabled Delay : Delay  DelayLength=1  ShowEnablePort=on  SampleTime=Ts
      settings: InputPortMap=u0,e6
  Gain{,1..5} (6 alike) : Gain  Gain=-1
  Gain6 : Gain
  Mux : Mux  Inputs=3
  Rate Limiter Dynamic : simulink/Discontinuities/Rate Limiter Dynamic
      settings: SourceProductName=Simulink
  Rate Limiter Dynamic1 : simulink/Discontinuities/Rate Limiter Dynamic
      settings: SourceProductName=Simulink
  Rate Limiter Dynamic2 : simulink/Discontinuities/Rate Limiter Dynamic
      settings: SourceProductName=Simulink
  Saturation Dynamic : simulink/Discontinuities/Saturation Dynamic  OutMin=[]  OutMax=[]  OutDataTypeStr=Inherit: Same as second input  OutDataType=fixdt(1, 16)  OutScaling=2^-10  DoSatur=off
  Saturation Dynamic1 : simulink/Discontinuities/Saturation Dynamic  OutMin=[]  OutMax=[]  OutDataTypeStr=Inherit: Same as second input  OutDataType=fixdt(1, 16)  OutScaling=2^-10  DoSatur=off
  Saturation Dynamic2 : simulink/Discontinuities/Saturation Dynamic  OutMin=[]  OutMax=[]  OutDataTypeStr=Inherit: Same as second input  OutDataType=fixdt(1, 16)  OutScaling=2^-10  DoSatur=off
  Subtract : Sum  Inputs=+-
  Switch : Switch  Criteria=u2 > Threshold
  Switch1 : Switch  Criteria=u2 > Threshold
  Switch2 : Switch  Criteria=u2 > Threshold
  dq_loc : Outport
  wires:
  Demux/1 -> Switch/3
  dq_setp/1 -> Demux/1
  new_cmd/1 -> Enabled Delay/2
  Digital Clock/1 -> Enabled Delay/1, Subtract/1
  Enabled Delay/1 -> Subtract/2
  Subtract/1 -> Compare To Constant/1
  Constant/1 -> Switch/1
  Gain/1 -> Rate Limiter Dynamic/3
  Switch/1 -> Saturation Dynamic/2
  Gain1/1 -> Saturation Dynamic/3
  Saturation Dynamic/1 -> Rate Limiter Dynamic/2
  Switch1/1 -> Saturation Dynamic1/2
  Gain3/1 -> Saturation Dynamic1/3
  Constant1/1 -> Switch1/1
  Demux/2 -> Switch1/3
  Gain2/1 -> Rate Limiter Dynamic1/3
  Saturation Dynamic1/1 -> Rate Limiter Dynamic1/2
  Bus Selector2/1 -> Rate Limiter Dynamic1/1, Gain2/1  "<max_acc_xy>"
  Bus Selector2/2 -> Saturation Dynamic1/1, Gain3/1  "<max_vel_xy>"
  Bus Selector3/1 -> Rate Limiter Dynamic2/1, Gain4/1  "<max_acc_theta>"
  Saturation Dynamic2/1 -> Rate Limiter Dynamic2/2
  base_conf/1 -> Bus Selector3/1, Bus Selector2/1, Bus Selector1/1
  Switch2/1 -> Saturation Dynamic2/2
  Constant2/1 -> Switch2/1
  Demux/3 -> Switch2/3
  Gain5/1 -> Saturation Dynamic2/3
  Gain4/1 -> Rate Limiter Dynamic2/3
  Compare To Constant/1 -> Gain6/1
  Bus Selector3/2 -> Saturation Dynamic2/1, Gain5/1  "<max_vel_theta>"
  Mux/1 -> dq_loc/1
  Rate Limiter Dynamic/1 -> Mux/1
  Rate Limiter Dynamic1/1 -> Mux/2
  Rate Limiter Dynamic2/1 -> Mux/3
  Bus Selector1/2 -> Saturation Dynamic/1, Gain1/1  "<max_vel_xy>"
  Bus Selector1/1 -> Rate Limiter Dynamic/1, Gain/1  "<max_acc_xy>"
  Gain6/1 -> Switch2/2, Switch1/2, Switch/2

== system ROPOD_4Wheel_Tdistkinb_cntr_Code_GEN/Ropod_Controller_No_ROS_EC/platform vel cntr ==
  ropod_kinmodel_pv : Inport
  sw_conf : Inport  Port=2
  disable : Inport  Port=3
  platform_dxdy_cntr_param : Inport  Port=4
  platform_dtheta_cntr_param : Inport  Port=5
  dqr_sp : Inport  Port=6
  dqr_loc : Inport  Port=7
  delta : Inport  Port=8
  ena_w : Inport  Port=9
  Inverse Kinematics 4SW : Subsystem
  Platorm Velocity controller : Subsystem
  Torque distribution : Subsystem
  dvarphi_sp : Outport
  varphi_tau_sp : Outport  Port=2
  wires:
  delta/1 -> Torque distribution/5(delta), Inverse Kinematics 4SW/3(delta)
  ena_w/1 -> Torque distribution/4(ena_w)
  sw_conf/1 -> Torque distribution/3(sw_conf)
  Torque distribution/1(varphi_tau_setp_out) -> varphi_tau_sp/1
  ropod_kinmodel_pv/1 -> Inverse Kinematics 4SW/1(param_in), Torque distribution/2(ropod_kinmodel_pv)
  Platorm Velocity controller/1(f_body_setp) -> Torque distribution/1(tau_body)
  disable/1 -> Platorm Velocity controller/1(reset_int)
  dqr_sp/1 -> Platorm Velocity controller/2(dqr_sp), Inverse Kinematics 4SW/2(dqr_sp)
  dqr_loc/1 -> Platorm Velocity controller/3(dqr_loc)
  Inverse Kinematics 4SW/1(wheel_vel_sp) -> dvarphi_sp/1
  platform_dxdy_cntr_param/1 -> Platorm Velocity controller/4(platform_dxdy_cntr_param)
  platform_dtheta_cntr_param/1 -> Platorm Velocity controller/5(platform_dtheta_cntr_param)

== system ROPOD_4Wheel_Tdistkinb_cntr_Code_GEN/Ropod_Controller_No_ROS_EC/wheel vel cntr ==
  disable : Inport
  platform_dxdy_cntr_param : Inport  Port=2
  dvarphi_sp : Inport  Port=3
  ena_w : Inport  Port=4
  dvarphi : Inport  Port=5
  Sum : Sum  Inputs=-+|
  Wheels Velocity controller : Subsystem
  varphi_tau_setp_out : Outport
  wires:
  Wheels Velocity controller/1(varphi_tau_setp) -> varphi_tau_setp_out/1
  ena_w/1 -> Wheels Velocity controller/2(ena_w)
  Sum/1 -> Wheels Velocity controller/1(dvarphi_error)
  dvarphi/1 -> Sum/1
  dvarphi_sp/1 -> Sum/2
  disable/1 -> Wheels Velocity controller/4(reset_int)
  platform_dxdy_cntr_param/1 -> Wheels Velocity controller/3(platform_dvarphi_cntr_param)

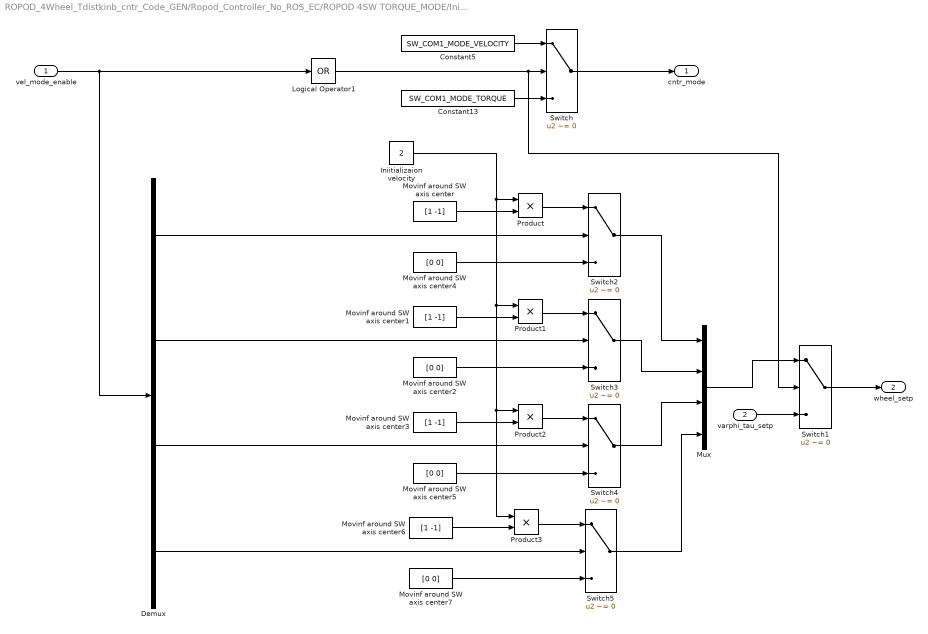
== system ROPOD_4Wheel_Tdistkinb_cntr_Code_GEN/Ropod_Controller_No_ROS_EC/ROPOD 4SW TORQUE_MODE/Initialization switch ==
  vel_mode_enable : Inport
  varphi_tau_setp : Inport  Port=2
  Constant13 : Constant  Value=SW_COM1_MODE_TORQUE
  Constant5 : Constant  Value=SW_COM1_MODE_VELOCITY
  Demux : Demux
  Iniitializaion velocity : Constant  Value=2
  Logical Operator1 : Logic  Operator=OR  Inputs=1  AllPortsSameDT=off  OutDataTypeStr=boolean
  Movinf around SW axis center{,1,3,6} (4 alike) : Constant  Value=[1 -1]
  Movinf around SW axis center{2,4..5,7} (4 alike) : Constant  Value=[0 0]
  Mux : Mux
  Product{,1..3} (4 alike) : Product
  Switch{,1..5} (6 alike) : Switch  Criteria=u2 ~= 0
  cntr_mode : Outport
  wheel_setp : Outport  Port=2
  wires:
  Constant13/1 -> Switch/3
  Constant5/1 -> Switch/1
  vel_mode_enable/1 -> Demux/1, Logical Operator1/1
  Switch/1 -> cntr_mode/1
  Logical Operator1/1 -> Switch1/2, Switch/2
  Movinf around SW axis center/1 -> Product/2
  Iniitializaion velocity/1 -> Product3/1, Product2/1, Product1/1, Product/1
  Product/1 -> Switch2/1
  Movinf around SW axis center4/1 -> Switch2/3
  Demux/1 -> Switch2/2
  Movinf around SW axis center2/1 -> Switch3/3
  Movinf around SW axis center1/1 -> Product1/2
  Demux/2 -> Switch3/2
  Product1/1 -> Switch3/1
  Movinf around SW axis center5/1 -> Switch4/3
  Movinf around SW axis center3/1 -> Product2/2
  Demux/3 -> Switch4/2
  Product2/1 -> Switch4/1
  Movinf around SW axis center7/1 -> Switch5/3
  Movinf around SW axis center6/1 -> Product3/2
  Demux/4 -> Switch5/2
  Product3/1 -> Switch5/1
  Switch2/1 -> Mux/1
  Switch3/1 -> Mux/2
  Switch4/1 -> Mux/3
  Switch5/1 -> Mux/4
  varphi_tau_setp/1 -> Switch1/3
  Mux/1 -> Switch1/1
  Switch1/1 -> wheel_setp/1

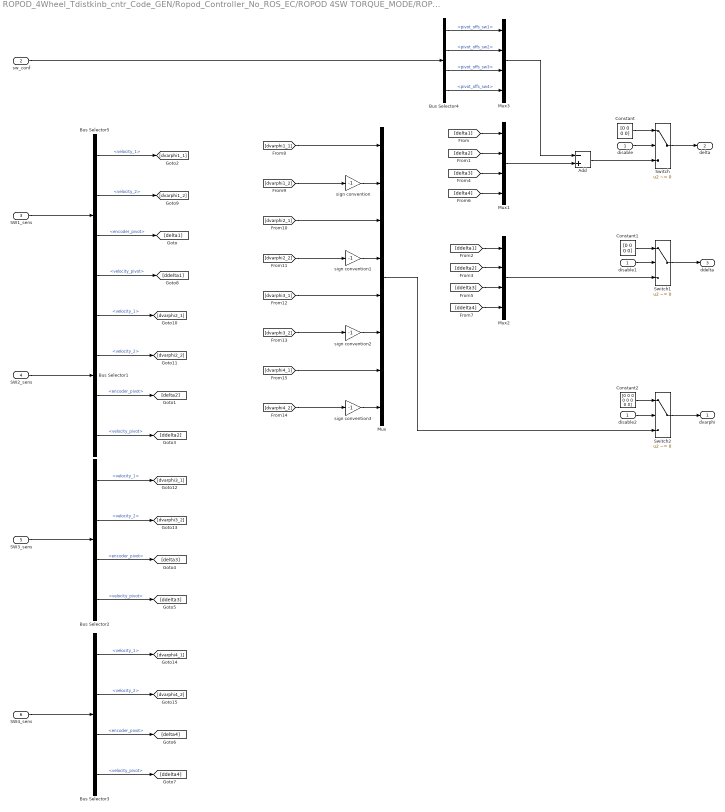
== system ROPOD_4Wheel_Tdistkinb_cntr_Code_GEN/Ropod_Controller_No_ROS_EC/ROPOD 4SW TORQUE_MODE/ROPOD_4Wheel_sens ==
  disable : Inport
  sw_conf : Inport  Port=2
  SW1_sens : Inport  Port=3
  SW2_sens : Inport  Port=4
  SW3_sens : Inport  Port=5
  SW4_sens : Inport  Port=6
  Add : Sum  Inputs=-+
  Bus Selector{1..3,5} (4 alike) : BusSelector  OutputSignals=velocity_1,velocity_2,encoder_pivot,velocity_pivot
  Bus Selector4 : BusSelector  OutputSignals=pivot_offs_sw1,pivot_offs_sw2,pivot_offs_sw3,pivot_offs_sw4
  Constant : Constant  Value=[0 0 0 0]
  Constant1 : Constant  Value=[0 0 0 0]
  Constant2 : Constant  Value=[0 0 0 0 0 0 0 0]
  Mux : Mux  Inputs=8
  Mux1 : Mux
  Mux2 : Mux
  Mux3 : Mux
  Switch : Switch  Criteria=u2 ~= 0
  Switch1 : Switch  Criteria=u2 ~= 0
  Switch2 : Switch  Criteria=u2 ~= 0
  disable1 : InportShadow
  disable2 : InportShadow
  sign convention{,1..3} (4 alike) : Gain  Gain=-1
  dvarphi : Outport
  delta : Outport  Port=2
  ddelta : Outport  Port=3
  wires:
  SW1_sens/1 -> Bus Selector5/1
  [delta1] -> Mux1/1
  [delta2] -> Mux1/2
  [ddelta2] -> Mux2/2
  [ddelta1] -> Mux2/1
  [delta3] -> Mux1/3
  [ddelta3] -> Mux2/3
  [delta4] -> Mux1/4
  [ddelta4] -> Mux2/4
  Mux1/1 -> Add/2
  Mux3/1 -> Add/1
  Bus Selector4/1 -> Mux3/1  "<pivot_offs_sw1>"
  Bus Selector4/2 -> Mux3/2  "<pivot_offs_sw2>"
  Bus Selector4/3 -> Mux3/3  "<pivot_offs_sw3>"
  Bus Selector4/4 -> Mux3/4  "<pivot_offs_sw4>"
  sign convention/1 -> Mux/2
  sign convention1/1 -> Mux/4
  sign convention2/1 -> Mux/6
  sign convention3/1 -> Mux/8
  Add/1 -> Switch/3
  Switch/1 -> delta/1
  disable/1 -> Switch/2
  Constant/1 -> Switch/1
  Switch1/1 -> ddelta/1
  Mux2/1 -> Switch1/3
  Constant1/1 -> Switch1/1
  disable1/1 -> Switch1/2
  disable2/1 -> Switch2/2
  Constant2/1 -> Switch2/1
  Mux/1 -> Switch2/3
  Switch2/1 -> dvarphi/1
  Bus Selector5/4 -> [ddelta1]  "<velocity_pivot>"
  Bus Selector5/2 -> [dvarphi1_2]  "<velocity_2>"
  sw_conf/1 -> Bus Selector4/1
  [dvarphi1_1] -> Mux/1
  [dvarphi1_2] -> sign convention/1
  [dvarphi2_1] -> Mux/3
  [dvarphi2_2] -> sign convention1/1
  [dvarphi3_1] -> Mux/5
  [dvarphi3_2] -> sign convention2/1
  [dvarphi4_1] -> Mux/7
  [dvarphi4_2] -> sign convention3/1
  Bus Selector5/1 -> [dvarphi1_1]  "<velocity_1>"
  Bus Selector5/3 -> [delta1]  "<encoder_pivot>"
  SW2_sens/1 -> Bus Selector1/1
  Bus Selector1/4 -> [ddelta2]  "<velocity_pivot>"
  Bus Selector1/1 -> [dvarphi2_1]  "<velocity_1>"
  Bus Selector1/3 -> [delta2]  "<encoder_pivot>"
  Bus Selector1/2 -> [dvarphi2_2]  "<velocity_2>"
  Bus Selector2/2 -> [dvarphi3_2]  "<velocity_2>"
  Bus Selector2/1 -> [dvarphi3_1]  "<velocity_1>"
  Bus Selector2/4 -> [ddelta3]  "<velocity_pivot>"
  SW3_sens/1 -> Bus Selector2/1
  Bus Selector2/3 -> [delta3]  "<encoder_pivot>"
  Bus Selector3/3 -> [delta4]  "<encoder_pivot>"
  SW4_sens/1 -> Bus Selector3/1
  Bus Selector3/4 -> [ddelta4]  "<velocity_pivot>"
  Bus Selector3/1 -> [dvarphi4_1]  "<velocity_1>"
  Bus Selector3/2 -> [dvarphi4_2]  "<velocity_2>"
